simulink model "AFMss_fp"  (R2016b)
settings: Solver=ode4  StartTime=0.0  StopTime=trun  FixedStep=Ts  RelTol=1e-5  EnableMultiTasking=on
PreLoadFcn:
  | VSS_CONTROL_MODE=1;
  | VSS_LINEAR_CONTROL=Simulink.Variant('VSS_CONTROL_MODE==1');
  | VSS_MPC_CONTROL=Simulink.Variant('VSS_CONTROL_MODE == 2');
  | 
  | 
  | VSS_STATE_DIRECT=Simulink.Variant('VSS_STATE_MODE==1');
  | VSS_STATE_OBS=Simulink.Variant('VSS_STATE_MODE==2');
  | VSS_STATE_DIST_OBS=Simulink.Variant('VSS_STATE_MODE==3');
  | VSS_STATE_MODE=1;
undefined symbols (not defined in the file): C_ydist, Ident_obs, PLANT, r, sim_struct, Ts, uss_0, VSS_OBS_DELUK_MODE, w, x0
libraries: cstblocks x2
settings Model: Creator=arnold  LastModifiedBy=arnold
settings DataIOCC: SaveFormat=Array  SaveOutput=off  SaveState=on  InspectSignalLogs=on  TimeSaveName=tout_ptos
settings OptimizationCC: LifeSpan=inf
settings DebuggingCC: SolverPrmCheckMsg=warning  SFUnexpectedBacktrackingDiag=warning  SFNoUnconditionalDefaultTransitionDiag=warning  SFExecutionAtInitializationDiag=none
settings HardwareCC: ProdBitPerPointer=32  ProdBitPerSizeT=32  ProdBitPerPtrDiffT=32  ProdLargestAtomicFloat=None  ProdIntDivRoundTo=Undefined  ProdEndianess=Unspecified  ProdWordSize=32  ProdHWDeviceType=32-bit Generic
settings ModelReferenceCC: PropagateSignalLabelsOutOfModel=off
settings GRTTargetCC: TargetLangStandard=C89/C90 (ANSI)  GeneratePreprocessorConditionals=Disable all
settings ConfigComp: CovMetricSettings=dw  CovHtmlReporting=on  CovSaveCumulativeToWorkspaceVar=on  CovSaveSingleToWorkspaceVar=on  CovExternalEMLEnable=off  CovSFcnEnable=off

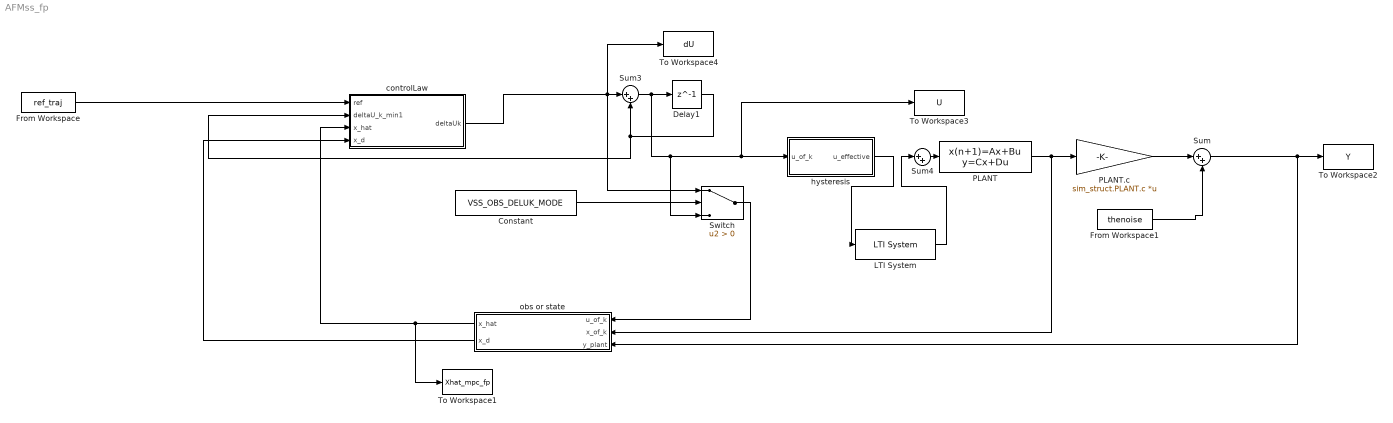
== system AFMss_fp ==
  Constant : Constant  Value=VSS_OBS_DELUK_MODE
  Delay1 : Delay  DelayLength=1  InitialCondition=uss_0  SampleTime=Ts
  From Workspace : FromWorkspace  VariableName=ref_traj  SampleTime=Ts
  From Workspace1 : FromWorkspace  VariableName=thenoise  SampleTime=Ts
  LTI System : cstblocks/LTI System  sys=sim_struct.gdrift  IC=[]
  PLANT : DiscreteStateSpace  A=PLANT.a  B=PLANT.b  C=eye(size(PLANT.b,1))  D=zeros(size(PLANT.b,1),1)  X0=x0  SampleTime=Ts
  PLANT.c : Gain  Gain=sim_struct.PLANT.c  Multiplication=Matrix(K*u)
  Sum : Sum  Inputs=|++
  Sum3 : Sum  Inputs=|++
  Sum4 : Sum  Inputs=|++
  Switch : Switch  Criteria=u2 > Threshold
  To Workspace1 : ToWorkspace  VariableName=Xhat_mpc_fp  SaveFormat=Timeseries  SampleTime=-1
      settings: Save2DSignal=2-D array (concatenate along first dimension)
  To Workspace2 : ToWorkspace  VariableName=Y  SaveFormat=Timeseries  SampleTime=-1
      settings: Save2DSignal=2-D array (concatenate along first dimension)
  To Workspace3 : ToWorkspace  VariableName=U  SaveFormat=Timeseries  SampleTime=-1
      settings: Save2DSignal=2-D array (concatenate along first dimension)
  To Workspace4 : ToWorkspace  VariableName=dU  SaveFormat=Timeseries  SampleTime=-1
      settings: Save2DSignal=2-D array (concatenate along first dimension)
  controlLaw : Subsystem
  hysteresis : Subsystem  Variant=on
  obs or state : Subsystem  Variant=on
  wires:
  PLANT/1 -> obs or state/2(x_of_k), PLANT.c/1
  Sum/1 -> obs or state/3(y_plant), To Workspace2/1
  obs or state/1(x_hat) -> controlLaw/3(x_hat), To Workspace1/1
  From Workspace1/1 -> Sum/2
  PLANT.c/1 -> Sum/1
  hysteresis/1(u_effective) -> LTI System/1
  Delay1/1 -> controlLaw/2(deltaU_k_min1), Sum3/2
  Sum3/1 -> Switch/3, To Workspace3/1, hysteresis/1(u_of_k), Delay1/1
  Sum4/1 -> PLANT/1
  Switch/1 -> obs or state/1(u_of_k)
  controlLaw/1(deltaUk) -> To Workspace4/1, Switch/1, Sum3/1
  From Workspace/1 -> controlLaw/1(ref)
  obs or state/2(x_d) -> controlLaw/4(x_d)
  Constant/1 -> Switch/2
  LTI System/1 -> Sum4/1

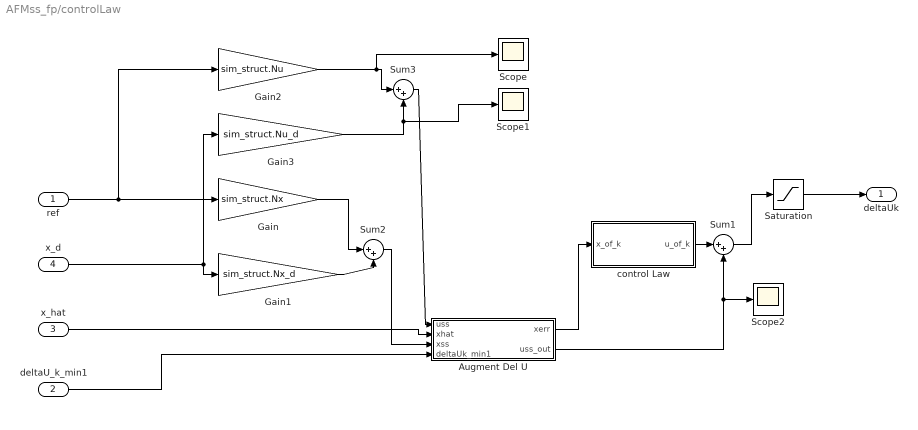
== system AFMss_fp/controlLaw ==
  ref : Inport
  deltaU_k_min1 : Inport  Port=2
  x_hat : Inport  Port=3
  x_d : Inport  Port=4
  Augment Del U : Subsystem  Variant=on
  Gain : Gain  Gain=sim_struct.Nx
  Gain1 : Gain  Gain=sim_struct.Nx_d
  Gain2 : Gain  Gain=sim_struct.Nu
  Gain3 : Gain  Gain=sim_struct.Nu_d
  Saturation : Saturate  UpperLimit=sim_struct.du_max  LowerLimit=-sim_struct.du_max
  Scope : Scope
  Scope1 : Scope
  Scope2 : Scope
  Sum1 : Sum  Inputs=|++
  Sum2 : Sum  Inputs=|++
  Sum3 : Sum  Inputs=|++
  control Law : Subsystem  Variant=on  OverrideUsingVariant=VSS_LINEAR_CONTROL
  deltaUk : Outport
  wires:
  deltaU_k_min1/1 -> Augment Del U/4(deltaUk_min1)
  Gain3/1 -> Scope1/1, Sum3/2
  x_hat/1 -> Augment Del U/2(xhat)
  Saturation/1 -> deltaUk/1
  Gain1/1 -> Sum2/2
  Sum1/1 -> Saturation/1
  Gain/1 -> Sum2/1
  Gain2/1 -> Scope/1, Sum3/1
  Sum2/1 -> Augment Del U/3(xss)
  control Law/1(u_of_k) -> Sum1/1
  ref/1 -> Gain/1, Gain2/1
  x_d/1 -> Gain3/1, Gain1/1
  Augment Del U/1(xerr) -> control Law/1(x_of_k)
  Augment Del U/2(uss_out) -> Scope2/1, Sum1/2
  Sum3/1 -> Augment Del U/1(uss)

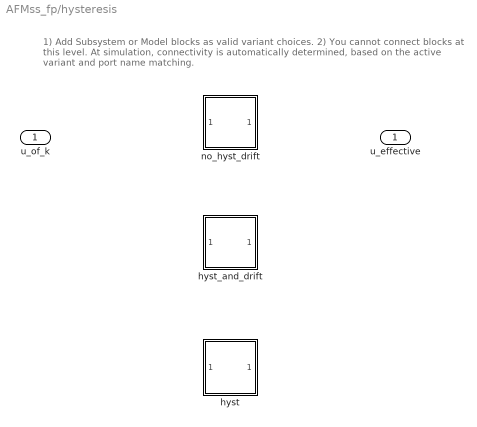
== system AFMss_fp/hysteresis ==
  note: 1) Add Subsystem or Model blocks as valid variant choices.
      | 2) You cannot connect blocks at this level. At simulation, connectivity is automatically
      | determined, based on the active variant and port name matching.
  u_of_k : Inport
  hyst : Subsystem  VariantControl=VSS_HYST_ONLY
  hyst_and_drift : Subsystem  VariantControl=VSS_HYST_AND_DRIFT
  no_hyst_drift : Subsystem  VariantControl=VSS_NO_HYST_NO_DRIFT
  u_effective : Outport

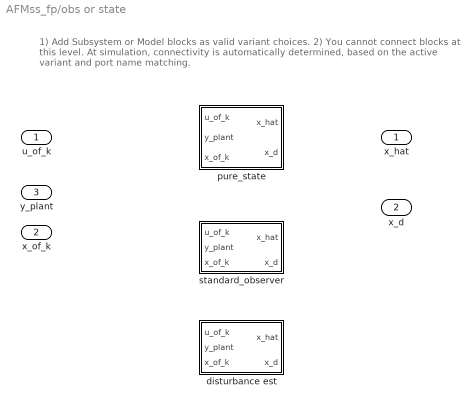
== system AFMss_fp/obs or state ==
  note: 1) Add Subsystem or Model blocks as valid variant choices.
      | 2) You cannot connect blocks at this level. At simulation, connectivity is automatically
      | determined, based on the active variant and port name matching.
  u_of_k : Inport
  x_of_k : Inport  Port=2
  y_plant : Inport  Port=3
  disturbance est : Subsystem  VariantControl=VSS_STATE_DIST_OBS
  pure_state : Subsystem  VariantControl=VSS_STATE_DIRECT
  standard_observer : Subsystem  VariantControl=VSS_STATE_OBS
  x_hat : Outport
  x_d : Outport  Port=2

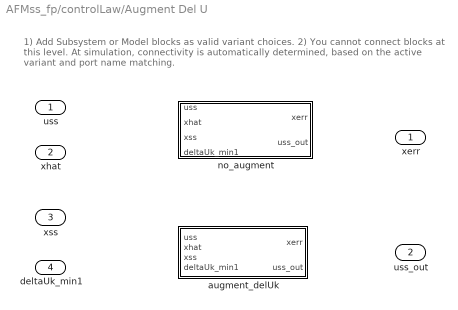
== system AFMss_fp/controlLaw/Augment Del U ==
  note: 1) Add Subsystem or Model blocks as valid variant choices.
      | 2) You cannot connect blocks at this level. At simulation, connectivity is automatically
      | determined, based on the active variant and port name matching.
  uss : Inport
  xhat : Inport  Port=2
  xss : Inport  Port=3
  deltaUk_min1 : Inport  Port=4
  augment_delUk : Subsystem  VariantControl=VSS_OBS_HAS_NO_DELUK
  no_augment : Subsystem  VariantControl=VSS_OBS_HAS_DELUK
  xerr : Outport
  uss_out : Outport  Port=2

== system AFMss_fp/controlLaw/control Law ==
  note: 1) Add Subsystem or Model blocks as valid variant choices.
      | 2) You cannot connect blocks at this level. At simulation, connectivity is automatically
      | determined, based on the active variant and port name matching.
  x_of_k : Inport
  linear_control : Subsystem  VariantControl=VSS_LINEAR_CONTROL
  mpc_control : Subsystem  VariantControl=VSS_MPC_CONTROL
  u_of_k : Outport

== system AFMss_fp/hysteresis/hyst ==
  u_of_k : Inport
  Delay : Delay  DelayLength=1  InitialCondition=zeros(length(r),1)
  MATLAB Function : MATLAB Function  TreatAsAtomicUnit=on
  u_effective : Outport
  wires:
  u_of_k/1 -> MATLAB Function/2(uk)
  MATLAB Function/1(xk) -> Delay/1
  Delay/1 -> MATLAB Function/1(xk_min1)
  MATLAB Function/2(H_uk) -> u_effective/1

== system AFMss_fp/hysteresis/hyst_and_drift ==
  u_of_k : Inport
  Delay : Delay  DelayLength=1  InitialCondition=zeros(length(r),1)
  LTI System1 : cstblocks/LTI System  sys=gdrift_inv  IC=x0_full
  MATLAB Function : MATLAB Function  TreatAsAtomicUnit=on
  u_effective : Outport
  wires:
  u_of_k/1 -> MATLAB Function/2(uk)
  MATLAB Function/2(H_uk) -> LTI System1/1
  MATLAB Function/1(xk) -> Delay/1
  Delay/1 -> MATLAB Function/1(xk_min1)
  LTI System1/1 -> u_effective/1

== system AFMss_fp/hysteresis/no_hyst_drift ==
  u_of_k : Inport
  u_effective : Outport
  wires:
  u_of_k/1 -> u_effective/1

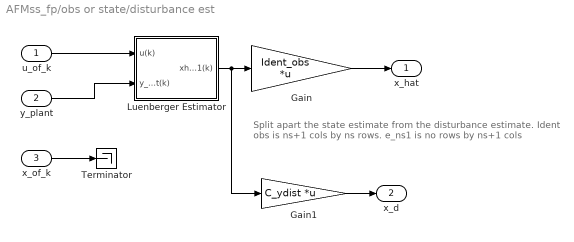
== system AFMss_fp/obs or state/disturbance est ==
  note: Split apart the state estimate from the disturbance estimate.
      | Ident obs is ns+1 cols by ns rows. e_ns1 is no rows by ns+1 cols
  u_of_k : Inport
  y_plant : Inport  Port=2
  x_of_k : Inport  Port=3
  Gain : Gain  Gain=Ident_obs  Multiplication=Matrix(K*u)
  Gain1 : Gain  Gain=C_ydist  Multiplication=Matrix(K*u)
  Luenberger Estimator : Subsystem  AncestorBlock=customLibFcns/Input Delay Luenberger Estimator
  Terminator : Terminator
  x_hat : Outport
  x_d : Outport  Port=2
  wires:
  u_of_k/1 -> Luenberger Estimator/1(u(k))
  x_of_k/1 -> Terminator/1
  Luenberger Estimator/1(xhat_1(k)) -> Gain1/1, Gain/1
  y_plant/1 -> Luenberger Estimator/2(y_plant(k))
  Gain/1 -> x_hat/1
  Gain1/1 -> x_d/1

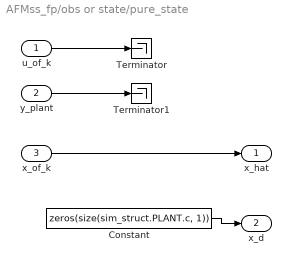
== system AFMss_fp/obs or state/pure_state ==
  u_of_k : Inport
  y_plant : Inport  Port=2
  x_of_k : Inport  Port=3
  Constant : Constant  Value=zeros(size(sim_struct.PLANT.c, 1))
  Terminator : Terminator
  Terminator1 : Terminator
  x_hat : Outport
  x_d : Outport  Port=2
  wires:
  y_plant/1 -> Terminator1/1
  u_of_k/1 -> Terminator/1
  x_of_k/1 -> x_hat/1
  Constant/1 -> x_d/1

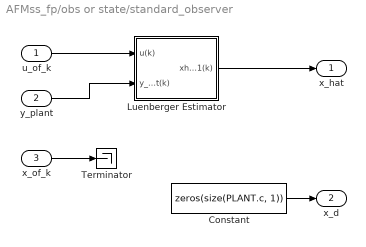
== system AFMss_fp/obs or state/standard_observer ==
  u_of_k : Inport
  y_plant : Inport  Port=2
  x_of_k : Inport  Port=3
  Constant : Constant  Value=zeros(size(PLANT.c, 1))
  Luenberger Estimator : Subsystem  AncestorBlock=customLibFcns/Input Delay Luenberger Estimator
  Terminator : Terminator
  x_hat : Outport
  x_d : Outport  Port=2
  wires:
  Luenberger Estimator/1(xhat_1(k)) -> x_hat/1
  y_plant/1 -> Luenberger Estimator/2(y_plant(k))
  u_of_k/1 -> Luenberger Estimator/1(u(k))
  x_of_k/1 -> Terminator/1
  Constant/1 -> x_d/1

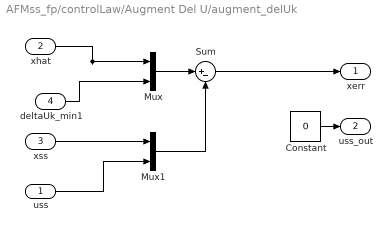
== system AFMss_fp/controlLaw/Augment Del U/augment_delUk ==
  uss : Inport
  xhat : Inport  Port=2
  xss : Inport  Port=3
  deltaUk_min1 : Inport  Port=4
  Constant : Constant  Value=0
  Mux : Mux  Inputs=2
  Mux1 : Mux  Inputs=2
  Sum : Sum  Inputs=|+-
  xerr : Outport
  uss_out : Outport  Port=2
  wires:
  Sum/1 -> xerr/1
  xhat/1 -> Mux/1
  deltaUk_min1/1 -> Mux/2
  uss/1 -> Mux1/2
  xss/1 -> Mux1/1
  Mux1/1 -> Sum/2
  Mux/1 -> Sum/1
  Constant/1 -> uss_out/1

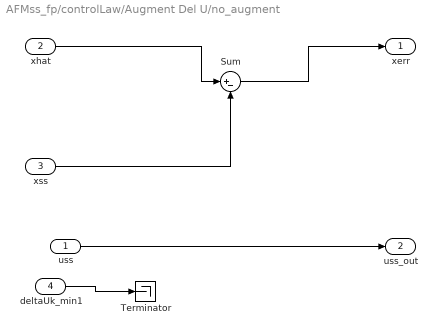
== system AFMss_fp/controlLaw/Augment Del U/no_augment ==
  uss : Inport
  xhat : Inport  Port=2
  xss : Inport  Port=3
  deltaUk_min1 : Inport  Port=4
  Sum : Sum  Inputs=|+-
  Terminator : Terminator
  xerr : Outport
  uss_out : Outport  Port=2
  wires:
  deltaUk_min1/1 -> Terminator/1
  xhat/1 -> Sum/1
  xss/1 -> Sum/2
  Sum/1 -> xerr/1
  uss/1 -> uss_out/1

== system AFMss_fp/controlLaw/control Law/linear_control ==
  x_of_k : Inport
  Gain1 : Gain  Gain=-sim_struct.K_lqr  Multiplication=Matrix(K*u)
  u_of_k : Outport
  wires:
  x_of_k/1 -> Gain1/1
  Gain1/1 -> u_of_k/1

== system AFMss_fp/controlLaw/control Law/mpc_control ==
  x_of_k : Inport
  Level-2 MATLAB S-Function : M-S-Function  FunctionName=mpcSolve  Parameters=sim_struct.mpcProb
  u_of_k : Outport
  wires:
  x_of_k/1 -> Level-2 MATLAB S-Function/1
  Level-2 MATLAB S-Function/1 -> u_of_k/1

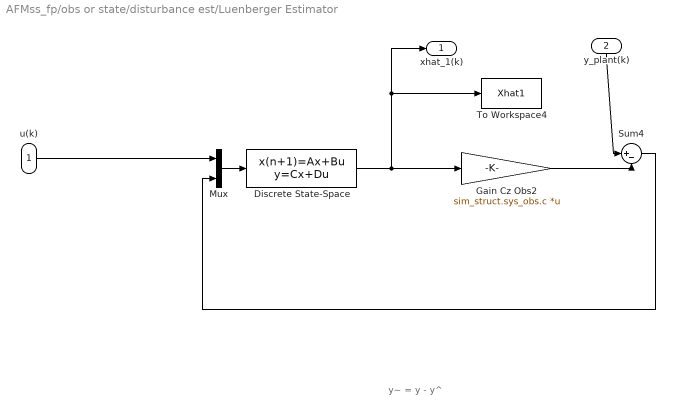
== system AFMss_fp/obs or state/disturbance est/Luenberger Estimator ==
  note: y~ = y - y^
  u(k) : Inport
  y_plant(k) : Inport  Port=2
  Discrete State-Space : DiscreteStateSpace  A=sim_struct.sys_obs.a  B=[sim_struct.sys_obs.b, sim_struct.L]  C=eye(length(sim_struct.sys_obs.b))  D=zeros(length(sim_struct.sys_obs.b), 2)  X0=sim_struct.x0_obs  SampleTime=Ts
  Gain Cz Obs2 : Gain  Gain=sim_struct.sys_obs.c  Multiplication=Matrix(K*u)
  Mux : Mux  Inputs=2
  Sum4 : Sum  Inputs=|+-
  To Workspace4 : ToWorkspace  VariableName=Xhat1  SaveFormat=Timeseries  SampleTime=-1
      settings: Save2DSignal=2-D array (concatenate along first dimension)
  xhat_1(k) : Outport
  wires:
  Sum4/1 -> Mux/2
  u(k)/1 -> Mux/1
  Mux/1 -> Discrete State-Space/1
  Discrete State-Space/1 -> Gain Cz Obs2/1, To Workspace4/1, xhat_1(k)/1
  Gain Cz Obs2/1 -> Sum4/2
  y_plant(k)/1 -> Sum4/1

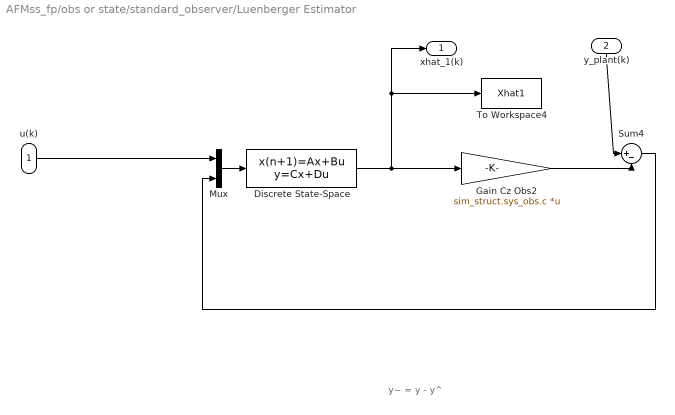
== system AFMss_fp/obs or state/standard_observer/Luenberger Estimator ==
  note: y~ = y - y^
  u(k) : Inport
  y_plant(k) : Inport  Port=2
  Discrete State-Space : DiscreteStateSpace  A=sim_struct.sys_obs.a  B=[sim_struct.sys_obs.b, sim_struct.L]  C=eye(length(sim_struct.sys_obs.b))  D=zeros(length(sim_struct.sys_obs.b), 2)  X0=sim_struct.x0_obs  SampleTime=Ts
  Gain Cz Obs2 : Gain  Gain=sim_struct.sys_obs.c  Multiplication=Matrix(K*u)
  Mux : Mux  Inputs=2
  Sum4 : Sum  Inputs=|+-
  To Workspace4 : ToWorkspace  VariableName=Xhat1  SaveFormat=Timeseries  SampleTime=-1
      settings: Save2DSignal=2-D array (concatenate along first dimension)
  xhat_1(k) : Outport
  wires:
  Sum4/1 -> Mux/2
  u(k)/1 -> Mux/1
  Mux/1 -> Discrete State-Space/1
  Discrete State-Space/1 -> Gain Cz Obs2/1, To Workspace4/1, xhat_1(k)/1
  Gain Cz Obs2/1 -> Sum4/2
  y_plant(k)/1 -> Sum4/1

== matlab function AFMss_fp/hysteresis/hyst/MATLAB Function ==
  data: xk output; xk_min1 input; uk input; H_uk output; r parameter; w parameter
function [xk, H_uk] = fcn(xk_min1, uk, r, w)

% n = length(r);
xk = r(:)*0;
    for j = 1:length(r)
        xk(j) = max(uk - r(j), min(uk+r(j), xk_min1(j)));
    end

    H_uk = w'*xk(:);

end

== matlab function AFMss_fp/hysteresis/hyst_and_drift/MATLAB Function ==
  data: xk output; xk_min1 input; uk input; H_uk output; r parameter; w parameter
function [xk, H_uk] = fcn(xk_min1, uk, r, w)

% n = length(r);
xk = r(:)*0;
    for j = 1:length(r)
        xk(j) = max(uk - r(j), min(uk+r(j), xk_min1(j)));
    end

    H_uk = w'*xk(:);

end
